simulink model "simulacion_ejemplo5_10"  (R2013a)
settings: Solver=ode45  StartTime=0.0  StopTime=10  FixedStep=0.01  RelTol=1e-3
values from neighbouring files (symbols this model uses):
  dr0 = 0    [ini_simulacion_ejemplo5_10.m]
  dtheta0 = 5*2*pi    (= 31.4159265359)    [ini_simulacion_ejemplo5_10.m]
  k1 = 2*0.5    (= 1)    [ini_simulacion_ejemplo5_10.m]
  k2 = 4*0.08    (= 0.32)    [ini_simulacion_ejemplo5_10.m]
  m = 10    [ini_simulacion_ejemplo5_10.m]
  omega = 5*2*pi    (= 31.4159265359)    [ini_simulacion_ejemplo5_10.m]
  r0 = 10    [ini_simulacion_ejemplo5_10.m]
  theta0 = 0    [ini_simulacion_ejemplo5_10.m]
settings Model: Creator=henry  LastModifiedBy=henry

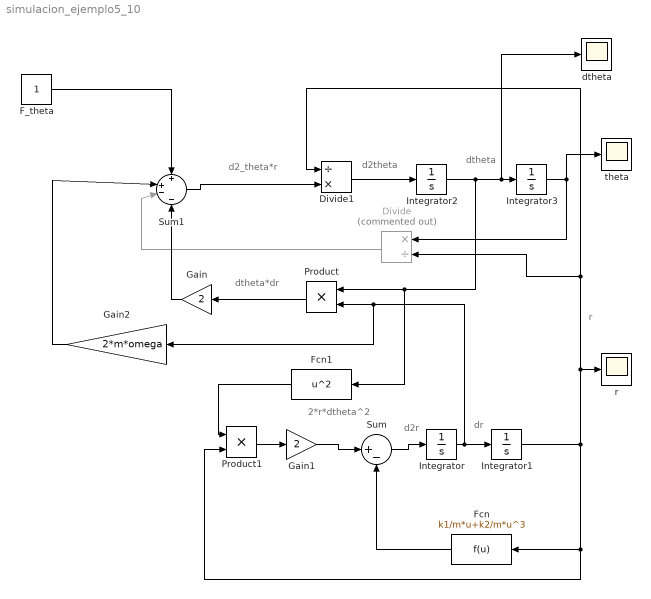
== system simulacion_ejemplo5_10 ==
  note: dtheta*dr
  note: 2*r*dtheta^2
  note: r
  note: dr
  note: d2r
  note: dtheta
  note: d2theta
  note: d2_theta*r
  Divide : Product  Commented=on  Inputs=*/
  Divide1 : Product  Inputs=/*
  F_theta : Constant
  Fcn : Fcn  Expr=k1/m*u+k2/m*u^3
  Fcn1 : Fcn  Expr=u^2
  Gain : Gain  Gain=2
  Gain1 : Gain  Gain=2
  Gain2 : Gain  Gain=2*m*omega
  Integrator : Integrator  InitialCondition=dr0
  Integrator1 : Integrator  InitialCondition=r0
  Integrator2 : Integrator  InitialCondition=dtheta0
  Integrator3 : Integrator  InitialCondition=theta0
  Product : Product
  Product1 : Product
  Sum : Sum  Inputs=|+-
  Sum1 : Sum  Inputs=+|+-|-
  dtheta : Scope
      settings: YMin=-11.15  YMax=-10.35  SaveName=ScopeData2
  r : Scope
      settings: YMin=208.25  YMax=211.25
  theta : Scope
      settings: YMin=-11.15  YMax=-10.35  MaxDataPoints=500000
  wires:
  Sum/1 -> Integrator/1
  Integrator/1 -> Integrator1/1, Gain2/1, Product/2
  Fcn/1 -> Sum/2
  Integrator3/1 -> Divide/1, theta/1
  Sum1/1 -> Divide1/2
  Divide1/1 -> Integrator2/1
  Integrator2/1 -> dtheta/1, Integrator3/1, Fcn1/1, Product/1
  Integrator1/1 -> r/1, Divide1/1, Divide/2, Fcn/1, Product1/2
  Divide/1 -> Sum1/3
  Product/1 -> Gain/1
  Gain/1 -> Sum1/4
  Gain1/1 -> Sum/1
  Product1/1 -> Gain1/1
  Fcn1/1 -> Product1/1
  F_theta/1 -> Sum1/1
  Gain2/1 -> Sum1/2
